simulink model "model"  (R2020b)
settings: Solver=VariableStepAuto  StartTime=0.0  StopTime=5  RelTol=1e-3
settings Model: Creator=64200047  LastModifiedBy=64200047

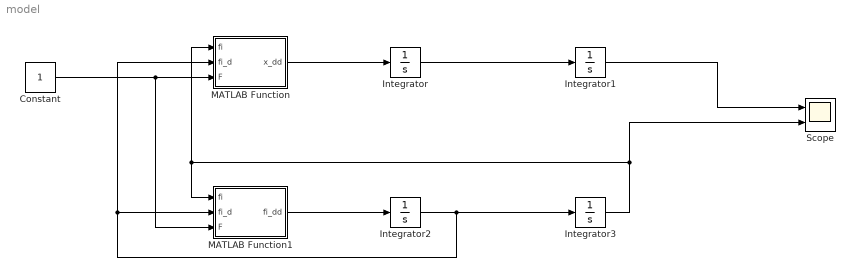
== system model ==
  Constant : Constant
  Integrator{,1..3} (4 alike) : Integrator
  MATLAB Function : MATLAB Function  TreatAsAtomicUnit=on
  MATLAB Function1 : MATLAB Function  TreatAsAtomicUnit=on
  Scope : Scope  NumInputPorts=2
  wires:
  MATLAB Function/1(x_dd) -> Integrator/1
  MATLAB Function1/1(fi_dd) -> Integrator2/1
  Integrator2/1 -> MATLAB Function/2(fi_d), MATLAB Function1/2(fi_d), Integrator3/1
  Integrator/1 -> Integrator1/1
  Constant/1 -> MATLAB Function1/3(F), MATLAB Function/3(F)
  Integrator3/1 -> Scope/2, MATLAB Function/1(fi), MATLAB Function1/1(fi)
  Integrator1/1 -> Scope/1

== matlab function model/MATLAB Function ==
  data: fi input; x_dd output; fi_d input; F input
function x_dd = fcn(fi, fi_d, F)
% x 

if ~exist('fi','var')
    fi = 0;
end
if ~exist('fi_d','var')
    fi_d = 0;
end

m1 = 2;
m2 = 0.31;
l = 0.5;

c1 = 1/(m1+m2);
k1 = +m2*l*sin(fi)*fi_d^2;
k2 = m2*l*cos(fi)*(cos(fi) + g*sin(fi));


x_dd = c1*(k1+k2+F);

== matlab function model/MATLAB Function1 ==
  data: fi input; fi_dd output; fi_d input; F input
function fi_dd = fcn(fi, fi_d, F)
% fi

m1 = 2;
m2 = 0.31;
l = 0.5;
g = 9.81;

c1 = 1/(-(m2*l*cos(fi))^2*1/(m1+m2) + m2*l^2);

k1 = -m2*l*cos(fi)*1/(m1+m2) * (F + m2*l*sin(fi)*fi_d^2) - m2*g*l*sin(fi);


    
fi_dd = c1*k1;
